simulink model "cruise_control_fechada"  (R2021b)
settings: Solver=FixedStepAuto  StartTime=0.0  StopTime=100  FixedStep=1e-3  RelTol=1e-3
values from neighbouring files (symbols this model uses):
  Kp = m/tau - b    [lab1parte3.m]
undefined symbols (not defined in the file or in its folder): b, bc, d, m, vr
settings Model: Creator=mmaximo  LastModifiedBy=buga
settings SolverCC: AlgebraicLoopSolver=TrustRegion
settings DebuggingCC: SFMachineParentedDataDiag=warning

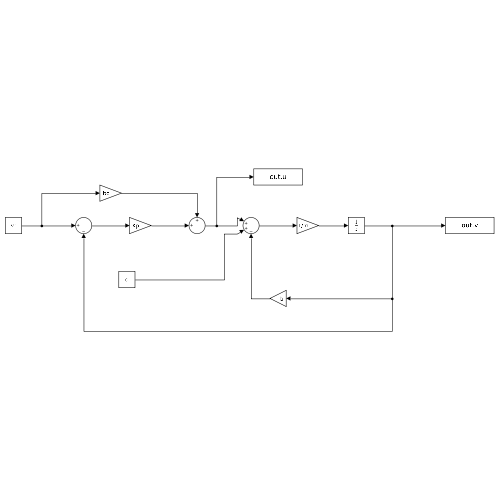
[thumbnail: Simulink's stored preview of the top-level diagram]
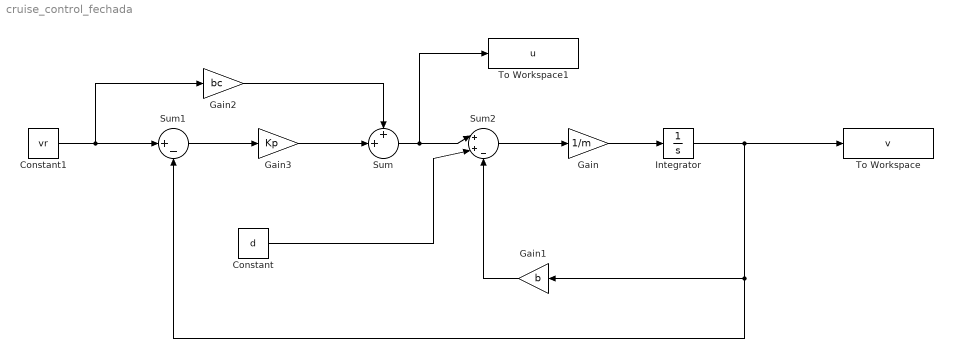
== system cruise_control_fechada ==
  Constant : Constant  Value=d
  Constant1 : Constant  Value=vr
  Gain : Gain  Gain=1/m
  Gain1 : Gain  Gain=b
  Gain2 : Gain  Gain=bc
  Gain3 : Gain  Gain=Kp
  Integrator : Integrator
  Sum : Sum  Inputs=++|
  Sum1 : Sum  Inputs=|+-
  Sum2 : Sum  Inputs=|++-
  To Workspace : ToWorkspace  VariableName=v  SaveFormat=Structure With Time  SampleTime=-1
  To Workspace1 : ToWorkspace  VariableName=u  SaveFormat=Structure With Time  SampleTime=-1
  wires:
  Gain3/1 -> Sum/2
  Sum1/1 -> Gain3/1
  Gain2/1 -> Sum/1
  Constant1/1 -> Gain2/1, Sum1/1
  Gain/1 -> Integrator/1
  Gain1/1 -> Sum2/3
  Integrator/1 -> To Workspace/1, Gain1/1, Sum1/2
  Constant/1 -> Sum2/2
  Sum/1 -> To Workspace1/1, Sum2/1
  Sum2/1 -> Gain/1
